simulink model "shiftregisterTut"  (R2013b)
settings: Solver=VariableStepDiscrete  StartTime=0.0  StopTime=5e-3  FixedStep=1e-3  MaxStep=100e-3  RelTol=1e-3
StopFcn:
  | run('spiBitBanging_process.m')
model workspace (MAT data in the model file):
  Ts = 1e-06
  periSam = 20
libraries: simulink x8, embdlinuxlib x4, dspswit3 x2, simulink_extras x2, powerlib_meascontrol x1, dspsnks4 x1
settings Model: PauseTimes=1.8  NumberOfSteps=100  SnapshotBufferSize=10000  SnapshotInterval=100  Creator=mainster  LastModifiedBy=mainster
settings ConfigurationSet: Description=SimMechanics 2G

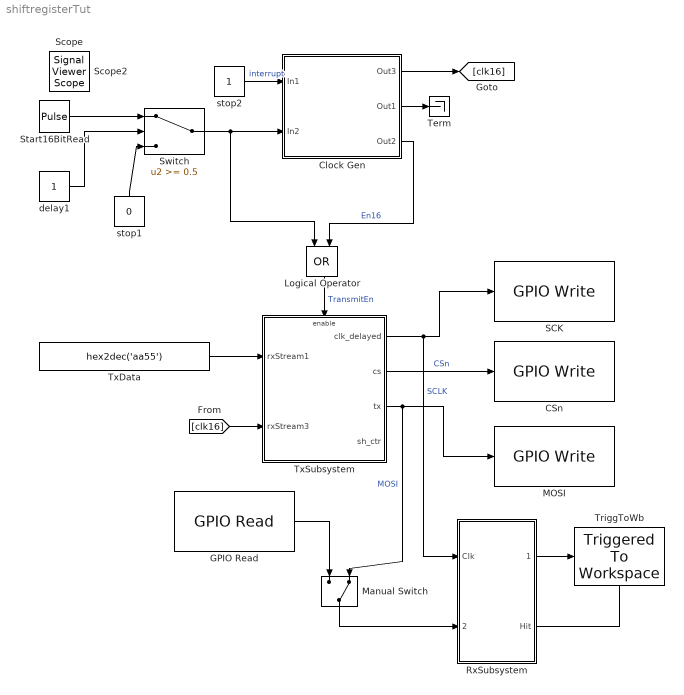
== system shiftregisterTut ==
  CSn : embdlinuxlib/GPIO Write  board=Model B Rev2  gpio=8  direction=Output  blockPlatform=Raspberry Pi
  Clock Gen : Subsystem
  GPIO Read : embdlinuxlib/GPIO Read  board=Model B Rev2  gpio=9  internalResistor=Off  sampleTime=Ts  direction=Input  blockPlatform=Raspberry Pi
  Logical Operator : Logic  Operator=OR  AllPortsSameDT=off  OutDataTypeStr=boolean
  MOSI : embdlinuxlib/GPIO Write  board=Model B Rev2  gpio=10  direction=Output  blockPlatform=Raspberry Pi
  Manual Switch : ManualSwitch  CurrentSetting=0
  RxSubsystem : Subsystem  InitFcn=filenameCtr=0;
  SCK : embdlinuxlib/GPIO Write  board=Model B Rev2  gpio=11  direction=Output  blockPlatform=Raspberry Pi
  Start16BitRead : DiscretePulseGenerator  Period=1000  PulseWidth=20  PhaseDelay=10  SampleTime=Ts
  Switch : Switch  Threshold=0.5
  Term : Terminator
  TriggToWb : dspsnks4/Triggered To Workspace  TriggerType=Rising edge  VariableName=RxDataRaw3  Buffer=1000  Save2DMode=2-D array (concatenate along first dimension)
      settings: FixptAsFi=off
  TxData : Constant  Value=hex2dec('aa55')  OutDataTypeStr=uint16  SampleTime=Ts
  TxSubsystem : Subsystem
      settings: PropExecContextOutsideSubsystem=on
  delay1 : Constant  SampleTime=Ts
  stop1 : Constant  Value=0  OutDataTypeStr=Inherit: Inherit via back propagation  SampleTime=Ts
  stop2 : Constant  OutDataTypeStr=Inherit: Inherit via back propagation  SampleTime=Ts
  Scope : SignalViewerScope  IOType=viewer  RefreshTime=0.035000
  Scope2 : SignalViewerScope  IOType=viewer  RefreshTime=0.035000
  wires:
  stop2/1 -> Clock Gen/1(In1)  "interrupt"
  Clock Gen/1(Out3) -> [clk16]
  Clock Gen/2(Out1) -> Term/1
  [clk16] -> TxSubsystem/2(rxStream3)
  Logical Operator/1 -> TxSubsystem/Enable  "TransmitEn"
  Clock Gen/3(Out2) -> Logical Operator/2  "En16"
  TxData/1 -> TxSubsystem/1(rxStream1)
  delay1/1 -> Switch/2
  stop1/1 -> Switch/3
  Start16BitRead/1 -> Switch/1
  Switch/1 -> Logical Operator/1, Clock Gen/2(In2)
  TxSubsystem/1(clk_delayed) -> RxSubsystem/1(Clk), SCK/1  "SCLK"
  TxSubsystem/3(tx) -> MOSI/1, Manual Switch/2  "MOSI"
  TxSubsystem/2(cs) -> CSn/1  "CSn"
  Manual Switch/1 -> RxSubsystem/2(sData_In)
  RxSubsystem/1(pData_Out) -> TriggToWb/1
  RxSubsystem/2(Hit) -> TriggToWb/Trigger
  GPIO Read/1 -> Manual Switch/1

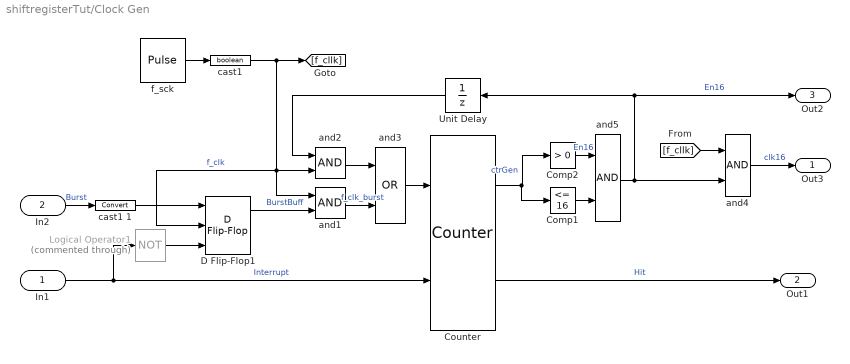
== system shiftregisterTut/Clock Gen ==
  In1 : Inport
  In2 : Inport  Port=2
  Comp1 : simulink/Logic and Bit Operations/Compare To Constant  relop=<=  const=16  OutDataTypeStr=boolean
  Comp2 : simulink/Logic and Bit Operations/Compare To Constant  relop=>  const=0  OutDataTypeStr=boolean
  Counter : dspswit3/Counter  Direction=Up  CountEvent=Rising edge  CounterSize=User defined  MaxCount=16  InitialCount=0  Output=Count and Hit  HitValue=periSam/4  ResetInput=on  SamplesPerFrame=1  Ts=1  CntDtype=double  HitDtype=Logical
  D Flip-Flop1 : simulink_extras/Flip Flops/D Flip-Flop
  Logical Operator1 : Logic  Commented=through  Operator=NOT  IconShape=distinctive  AllPortsSameDT=off  OutDataTypeStr=boolean
  Unit Delay : UnitDelay  SampleTime=-1
  and{1..2,4..5} (4 alike) : Logic  AllPortsSameDT=off  OutDataTypeStr=boolean
      settings: AttributesFormatString=%<Tag>
  and3 : Logic  Operator=OR  AllPortsSameDT=off  OutDataTypeStr=boolean
      settings: AttributesFormatString=%<Tag>
  "cast1 " : DataTypeConversion  OutDataTypeStr=boolean
  cast1 1 : DataTypeConversion
  f_sck : DiscretePulseGenerator  Period=periSam  PulseWidth=periSam/2  SampleTime=Ts
      settings: AttributesFormatString=|
      | Period =%<Period>
      | sTime=%<SampleTime>
      | Delay=%<PhaseDelay>
  Out3 : Outport
  Out1 : Outport  Port=2
  Out2 : Outport  Port=3
  wires:
  "cast1 "/1 -> and1/1, D Flip-Flop1/2, and2/2, [f_cllk]  "f_clk"
  f_sck/1 -> "cast1 "/1
  In1/1 -> Logical Operator1/1, Counter/2  "Interrupt"
  and3/1 -> Counter/1
  and4/1 -> Out3/1  "clk16"
  and1/1 -> and3/2  "f_clk_burst"
  and2/1 -> and3/1
  Unit Delay/1 -> and2/1
  Counter/2 -> Out1/1  "Hit"
  [f_cllk] -> and4/1
  Counter/1 -> Comp1/1, Comp2/1  "ctrGen"
  and5/1 -> Unit Delay/1, Out2/1, and4/2  "En16"
  Comp2/1 -> and5/1  "En16"
  Comp1/1 -> and5/2
  cast1 1/1 -> D Flip-Flop1/1
  Logical Operator1/1 -> D Flip-Flop1/3
  In2/1 -> cast1 1/1  "Burst"
  D Flip-Flop1/1 -> and1/2  "BurstBuff"

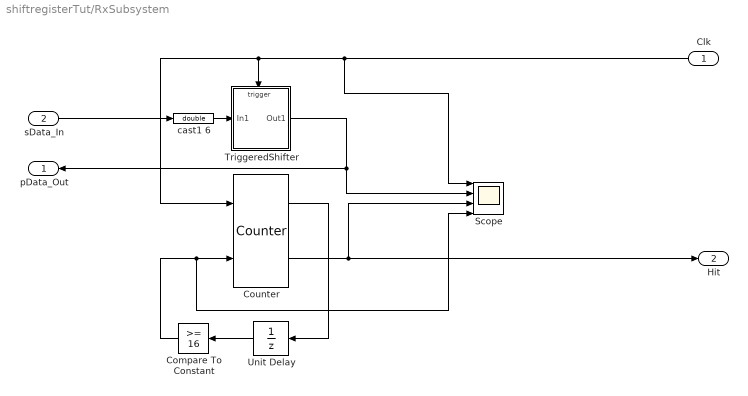
== system shiftregisterTut/RxSubsystem ==
  Clk : Inport
  sData_In : Inport  Port=2
  Compare To Constant : simulink/Logic and Bit Operations/Compare To Constant  relop=>=  const=16  OutDataTypeStr=boolean
  Counter : dspswit3/Counter  Direction=Up  CountEvent=Rising edge  CounterSize=User defined  MaxCount=17  InitialCount=0  Output=Count and Hit  HitValue=16  ResetInput=on  SamplesPerFrame=1  Ts=1  CntDtype=double  HitDtype=Logical
  Scope : Scope  NumInputPorts=4
      settings: ShowLegends=on  TimeRange=0.0004  YMin=-0.2~-0.2~-1~-0.2  YMax=1.2~1.2~1~1.2
  TriggeredShifter : Subsystem
      settings: RTWSystemCode=Inline
  Unit Delay : UnitDelay  SampleTime=-1
  cast1 6 : DataTypeConversion  OutDataTypeStr=double  LockScale=on
  pData_Out : Outport
  Hit : Outport  Port=2
  wires:
  TriggeredShifter/1(Out1) -> Scope/2, pData_Out/1
  Clk/1 -> Counter/1, TriggeredShifter/Trigger, Scope/1
  Counter/1 -> Unit Delay/1
  Compare To Constant/1 -> Scope/4, Counter/2
  Counter/2 -> Scope/3, Hit/1
  sData_In/1 -> cast1 6/1
  Unit Delay/1 -> Compare To Constant/1
  cast1 6/1 -> TriggeredShifter/1(In1)

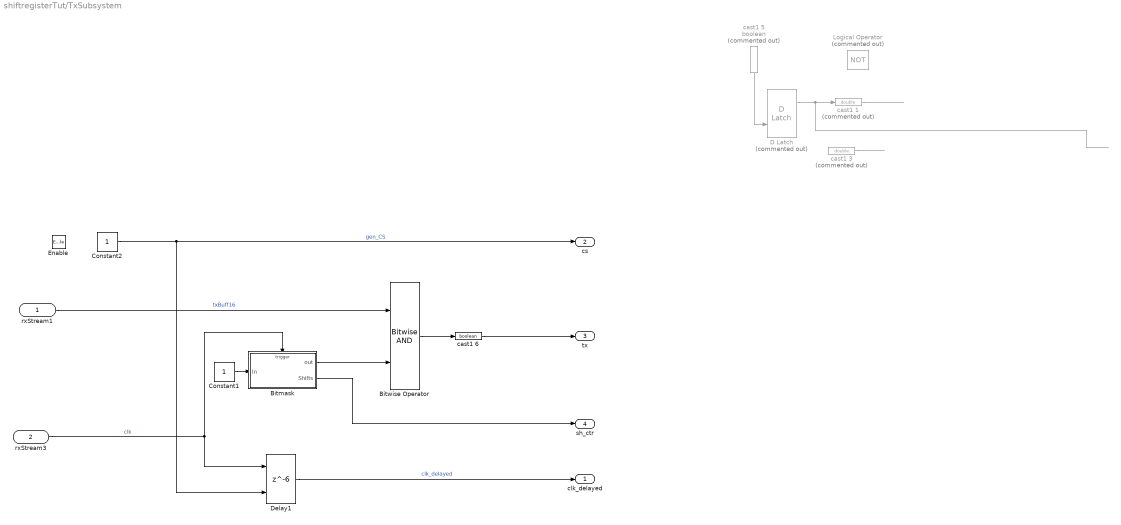
== system shiftregisterTut/TxSubsystem ==
  rxStream1 : Inport  OutDataTypeStr=uint16
  rxStream3 : Inport  Port=2
  Enable : EnablePort  StatesWhenEnabling=reset
  Bitmask : Subsystem  TreatAsAtomicUnit=on
  Bitwise Operator : simulink/Logic and Bit Operations/Bitwise Operator  logicop=AND  UseBitMask=off  NumInputPorts=2  BitMask=bin2dec('11011001')  BitMaskRealWorld=Stored Integer
  Constant1 : Constant
  Constant2 : Constant
  D Latch : simulink_extras/Flip Flops/D Latch  Commented=on
  Delay1 : Delay  DelayLength=6  InitialCondition=0  ExternalReset=Rising  InputProcessing=Inherited  SampleTime=Ts
      settings: InputPortMap=u0,r5
  Logical Operator : Logic  Commented=on  Operator=NOT  IconShape=distinctive  AllPortsSameDT=off  OutDataTypeStr=boolean
  cast1 1 : DataTypeConversion  Commented=on  OutDataTypeStr=double  LockScale=on
  cast1 3 : DataTypeConversion  Commented=on  OutDataTypeStr=double  LockScale=on
  cast1 5 : DataTypeConversion  Commented=on  OutDataTypeStr=boolean  LockScale=on
  cast1 6 : DataTypeConversion  OutDataTypeStr=boolean  LockScale=on
  clk_delayed : Outport  OutputWhenDisabled=reset  InitialOutput=0
  cs : Outport  Port=2  OutputWhenDisabled=reset  InitialOutput=1
  tx : Outport  Port=3  OutputWhenDisabled=reset  InitialOutput=1
  sh_ctr : Outport  Port=4  OutputWhenDisabled=reset  InitialOutput=1
  wires:
  Constant2/1 -> cs/1, Delay1/2  "gen_CS"
  rxStream1/1 -> Bitwise Operator/1  "txBuff16"
  rxStream3/1 -> Bitmask/Trigger, Delay1/1  "clk"
  Constant1/1 -> Bitmask/1(In)
  Bitmask/1(out) -> Bitwise Operator/2
  Delay1/1 -> clk_delayed/1  "clk_delayed"
  Bitwise Operator/1 -> cast1 6/1
  ? -> ?  "gen_CS"
  ? -> cast1 5/1  "txBuff16"
  ? -> ?  "clk"
  ? -> ?
  ? -> cast1 3/1
  cast1 1/1 -> ?
  cast1 3/1 -> ?
  D Latch/1 -> cast1 1/1
  cast1 5/1 -> D Latch/2
  ? -> D Latch/1
  Bitmask/2(Shifts) -> sh_ctr/1
  cast1 6/1 -> tx/1

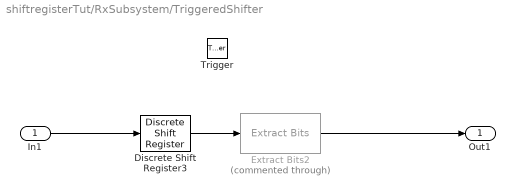
== system shiftregisterTut/RxSubsystem/TriggeredShifter ==
  In1 : Inport
  Trigger : TriggerPort  PortDimensions=1
  Discrete Shift Register3 : powerlib_meascontrol/Additional Components/Discrete Shift Register  NSamples=16  InitialValue=0  Ts=-1
  Extract Bits2 : simulink/Logic and Bit Operations/Extract Bits  Commented=through  bitsToExtract=Range of bits  numBits=8  bitIdxRange=1  outScalingMode=Treat bit field as an integer
  Out1 : Outport
  wires:
  Discrete Shift Register3/1 -> Extract Bits2/1
  Extract Bits2/1 -> Out1/1
  In1/1 -> Discrete Shift Register3/1

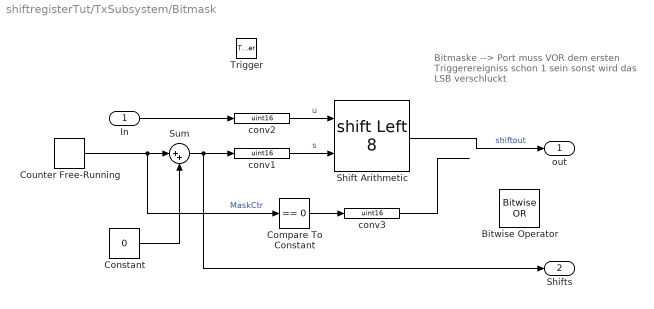
== system shiftregisterTut/TxSubsystem/Bitmask ==
  note: Bitmaske --> Port muss VOR dem ersten
      | Triggerereigniss schon 1 sein sonst wird
      | das LSB verschluckt
  In : Inport
  Trigger : TriggerPort  PortDimensions=1
  Bitwise Operator : simulink/Logic and Bit Operations/Bitwise Operator  logicop=OR  UseBitMask=off  NumInputPorts=2  BitMask=2  BitMaskRealWorld=Stored Integer
  Compare To Constant : simulink/Logic and Bit Operations/Compare To Constant  relop===  const=0  OutDataTypeStr=uint8
  Constant : Constant  Value=0  SampleTime=-1
  Counter Free-Running : simulink/Sources/Counter Free-Running  NumBits=14  tsamp=-1
  Shift Arithmetic : ArithShift  BitShiftNumberSource=Input port  BitShiftNumber=8  BitShiftDirection=Left  DiagnosticForOORShift=Error
      settings: InputPortMap=u0,p1
  Sum : Sum  Inputs=|++
  conv1 : DataTypeConversion  OutDataTypeStr=uint16
  conv2 : DataTypeConversion  OutDataTypeStr=uint16
  conv3 : DataTypeConversion  OutDataTypeStr=uint16
  out : Outport  InitialOutput=[1]
  Shifts : Outport  Port=2
  wires:
  Shift Arithmetic/1 -> out/1  "shiftout"
  In/1 -> conv2/1
  Sum/1 -> Shifts/1, conv1/1
  Constant/1 -> Sum/2
  conv1/1 -> Shift Arithmetic/2  "s"
  conv2/1 -> Shift Arithmetic/1  "u"
  Counter Free-Running/1 -> Compare To Constant/1, Sum/1  "MaskCtr"
  Compare To Constant/1 -> conv3/1
  conv3/1 -> ?
